simulink model "pwm2_process"  (Simulink 3.00)
libraries: modellib x1, mathlib x1

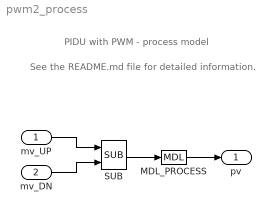
== system pwm2_process ==
  note: See the README.md file for detailed information.
  note: PIDU with PWM - process model
  mv_UP : Inport  Port=1
  mv_DN : Inport  Port=2
  MDL_PROCESS : modellib/MDL  k0=10  del=0  tau1=8  tau2=5  nmax=100
  SUB : mathlib/SUB
  pv : Outport  Port=1
  wires:
  MDL_PROCESS/1 -> pv/1
  SUB/1 -> MDL_PROCESS/1
  mv_DN/1 -> SUB/2
  mv_UP/1 -> SUB/1
